simulink model "Closed_Loop_Neural_Attitude_plant_MRAC_for_roll_good"  (R2018b)
settings: Solver=VariableStepAuto  StartTime=0.0  StopTime=500  FixedStep=0.0001  RelTol=1e3  EnableMultiTasking=on
undefined symbols (not defined in the file): DiscIntNeverNeededParam
libraries: dspmtrx3 x6, neural x3, vrlib x2, sharedutil x1
CloseFcn:
  | rtwprivate ssgencode ModelCloseRequest controller
settings Model: Creator=acer  LastModifiedBy=the other guy
settings SolverCC: ZeroCrossControl=DisableAll  AutoInsertRateTranBlk=on
settings DataIOCC: LimitDataPoints=on  SaveFormat=Array  SignalLoggingSaveFormat=ModelDataLogs
settings OptimizationCC: ExpressionDepthLimit=2147483647  LifeSpan=inf
settings DebuggingCC: SaveWithParameterizedLinksMsg=none  UnderspecifiedInitializationDetection=Classic  MergeDetectMultiDrivingBlocksExec=none  SolverPrmCheckMsg=warning  FcnCallInpInsideContextMsg=warning  StateNameClashWarn=warning  SFUnexpectedBacktrackingDiag=warning  SFNoUnconditionalDefaultTransitionDiag=warning  SFExecutionAtInitializationDiag=none
settings HardwareCC: ProdBitPerPointer=32  ProdBitPerSizeT=32  ProdBitPerPtrDiffT=32  ProdLargestAtomicFloat=None  ProdIntDivRoundTo=Undefined  ProdEndianess=Unspecified  ProdWordSize=32  ProdHWDeviceType=32-bit Generic
settings ModelReferenceCC: PropagateSignalLabelsOutOfModel=off
settings SFSimCC: SimUseLocalCustomCode=off
settings RTWCC: RTWUseLocalCustomCode=off
settings CodeAppCC: StateflowObjectComments=on
settings GRTTargetCC: TargetLangStandard=C89/C90 (ANSI)  GeneratePreprocessorConditionals=Disable all  CombineOutputUpdateFcns=off  GRTInterface=on
settings ConfigComp: CovMetricSettings=dw  CovHtmlReporting=on  CovSaveCumulativeToWorkspaceVar=on  CovSaveSingleToWorkspaceVar=on  CovExternalEMLEnable=off

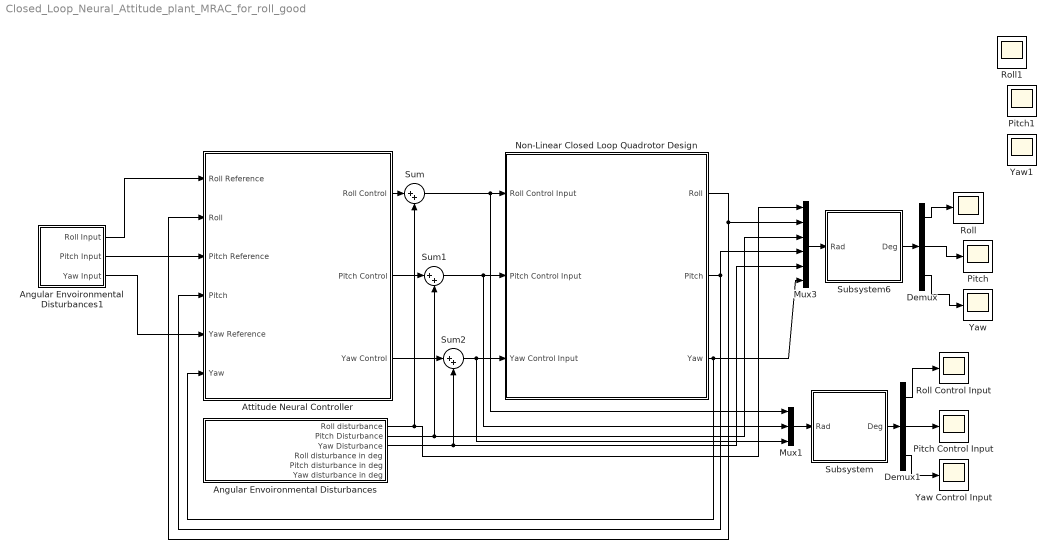
== system Closed_Loop_Neural_Attitude_plant_MRAC_for_roll_good ==
  Angular Envoironmental Disturbances : Subsystem
  Angular Envoironmental Disturbances1 : Subsystem
  Attitude Neural Controller : Subsystem
  Demux : Demux  Outputs=[2,2,2]
  Demux1 : Demux  Outputs=3
  Mux1 : Mux  Inputs=3
  Mux3 : Mux  Inputs=6
  Non-Linear Closed Loop Quadrotor Design : Subsystem
  Pitch : Scope
  Pitch Control Input : Scope
  Pitch1 : Scope
  Roll : Scope
  Roll Control Input : Scope
  Roll1 : Scope
  Subsystem : Subsystem
  Subsystem6 : Subsystem
  Sum : Sum  Inputs=|++
  Sum1 : Sum  Inputs=|++
  Sum2 : Sum  Inputs=|++
  Yaw : Scope
  Yaw Control Input : Scope
  Yaw1 : Scope
  wires:
  Non-Linear Closed Loop Quadrotor Design/1(Roll) -> Mux3/2, Attitude Neural Controller/2(Roll)
  Angular Envoironmental Disturbances1/1(Roll Input) -> Attitude Neural Controller/1(Roll Reference)
  Demux1/1 -> Roll Control Input/1
  Angular Envoironmental Disturbances1/2(Pitch Input) -> Attitude Neural Controller/3(Pitch Reference)
  Non-Linear Closed Loop Quadrotor Design/2(Pitch) -> Attitude Neural Controller/4(Pitch), Mux3/4
  Demux1/2 -> Pitch Control Input/1
  Sum1/1 -> Mux1/2, Non-Linear Closed Loop Quadrotor Design/2(Pitch Control Input)
  Sum/1 -> Mux1/1, Non-Linear Closed Loop Quadrotor Design/1(Roll Control Input)
  Sum2/1 -> Mux1/3, Non-Linear Closed Loop Quadrotor Design/3(Yaw Control Input)
  Non-Linear Closed Loop Quadrotor Design/3(Yaw) -> Attitude Neural Controller/6(Yaw), Mux3/6
  Angular Envoironmental Disturbances1/3(Yaw Input) -> Attitude Neural Controller/5(Yaw Reference)
  Demux1/3 -> Yaw Control Input/1
  Mux3/1 -> Subsystem6/1(Rad)
  Subsystem6/1(Deg) -> Demux/1
  Demux/2 -> Pitch/1
  Mux1/1 -> Subsystem/1(Rad)
  Subsystem/1(Deg) -> Demux1/1
  Attitude Neural Controller/3(Yaw Control) -> Sum2/1
  Attitude Neural Controller/2(Pitch Control) -> Sum1/1
  Attitude Neural Controller/1(Roll Control) -> Sum/1
  Demux/1 -> Roll/1
  Demux/3 -> Yaw/1
  Angular Envoironmental Disturbances/1(Roll disturbance) -> Mux3/1, Sum/2
  Angular Envoironmental Disturbances/2(Pitch Disturbance) -> Mux3/3, Sum1/2
  Angular Envoironmental Disturbances/3(Yaw Disturbance) -> Mux3/5, Sum2/2

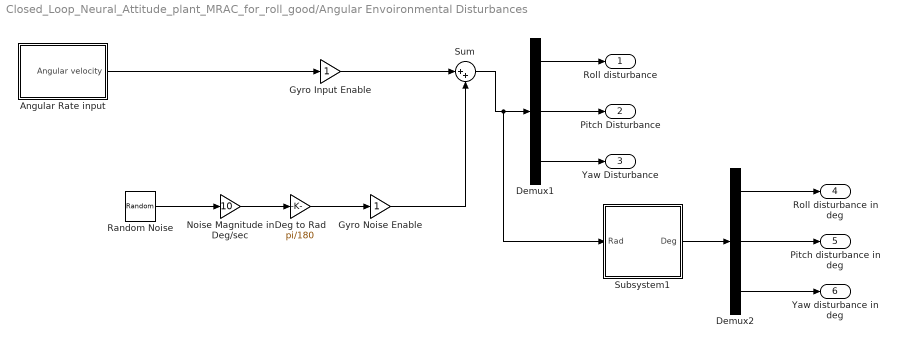
== system Closed_Loop_Neural_Attitude_plant_MRAC_for_roll_good/Angular Envoironmental Disturbances ==
  Angular Rate input : Subsystem
  Deg to Rad : Gain  Gain=pi/180
  Demux1 : Demux  Outputs=3
  Demux2 : Demux  Outputs=3
  Gyro Input Enable : Gain
  Gyro Noise Enable : Gain
  Noise Magnitude in Deg/sec : Gain  Gain=10
  Random Noise : RandomNumber  Variance=0.25  SampleTime=0
  Subsystem1 : Subsystem
  Sum : Sum  Inputs=|++
  Roll disturbance : Outport
  Pitch Disturbance : Outport  Port=2
  Yaw Disturbance : Outport  Port=3
  Roll disturbance in deg : Outport  Port=4
  Pitch disturbance in deg : Outport  Port=5
  Yaw disturbance in deg : Outport  Port=6
  wires:
  Random Noise/1 -> Noise Magnitude in Deg/sec/1
  Sum/1 -> Subsystem1/1(Rad), Demux1/1
  Gyro Noise Enable/1 -> Sum/2
  Angular Rate input/1(Angular velocity) -> Gyro Input Enable/1
  Deg to Rad/1 -> Gyro Noise Enable/1
  Noise Magnitude in Deg/sec/1 -> Deg to Rad/1
  Gyro Input Enable/1 -> Sum/1
  Demux1/1 -> Roll disturbance/1
  Demux1/2 -> Pitch Disturbance/1
  Demux1/3 -> Yaw Disturbance/1
  Subsystem1/1(Deg) -> Demux2/1
  Demux2/1 -> Roll disturbance in deg/1
  Demux2/3 -> Yaw disturbance in deg/1
  Demux2/2 -> Pitch disturbance in deg/1

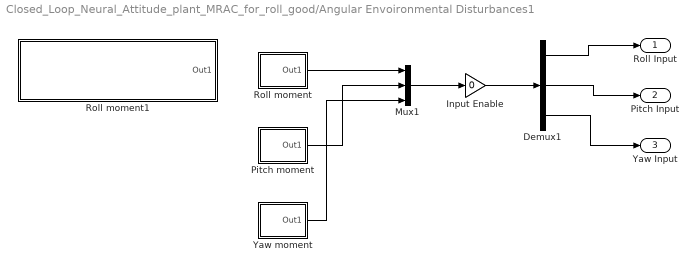
== system Closed_Loop_Neural_Attitude_plant_MRAC_for_roll_good/Angular Envoironmental Disturbances1 ==
  Demux1 : Demux  Outputs=3
  Input Enable : Gain  Gain=0
  Mux1 : Mux  Inputs=3
  Pitch moment : Subsystem  mask(timed input){t=[0 100 100 500], u=[0 0 25 25]*pi/180}
      mask prompts: t "time values:"; u "input values"
      mask Display: plot(t,u)
  Roll moment : Subsystem  mask(timed input){t=[0 200 200 500], u=[0 0 20 20]*pi/180}
      mask prompts: t "time values:"; u "input values"
      mask Display: plot(t,u)
  Roll moment1 : Subsystem  mask(timed input){t=[0 1 1 2 2 3 3 4 4 6 6 8 8 10 10 12 12 15 15 18 18 21 21 24 24 25 25 26.5 26.5 28 28 29.5 29.5 31 31 32 32 33 33 34 34 35 35 37.5, 37.5 40 40 42.5 42.5 45 45 47.5 47.5 48 48 48.5 48.5 49 49 49.5 49.5 50]*100, u=[-60 -60 60 60 60 60 -60 -60 40 40 -40 -40 -40 -40 40 40 -10 -10 10 10 10 10 -10 -10 0 0 -25 -25 25 25 25 25 -25 -25 70 70 -70 -70 -70 -70 70 70 0 0 -5 -5 5 5 5 5 -5 -5 50 50 -50 -50 -50 -50 50 50 0 0]*pi/180}
      mask prompts: t "time values:"; u "input values"
      mask Display: plot(t,u)
  Yaw moment : Subsystem  mask(timed input){t=[0 300 300 500], u=[0 0 10 10]*pi/180}
      mask prompts: t "time values:"; u "input values"
      mask Display: plot(t,u)
  Roll Input : Outport
  Pitch Input : Outport  Port=2
  Yaw Input : Outport  Port=3
  wires:
  Roll moment/1(Out1) -> Mux1/1
  Demux1/1 -> Roll Input/1
  Demux1/2 -> Pitch Input/1
  Demux1/3 -> Yaw Input/1
  Input Enable/1 -> Demux1/1
  Mux1/1 -> Input Enable/1
  Pitch moment/1(Out1) -> Mux1/2
  Yaw moment/1(Out1) -> Mux1/3

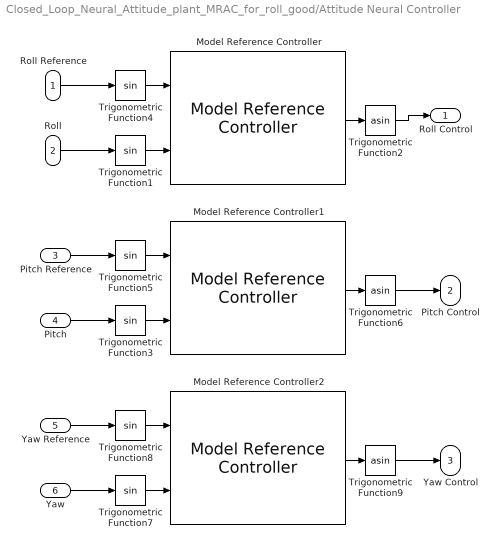
== system Closed_Loop_Neural_Attitude_plant_MRAC_for_roll_good/Attitude Neural Controller ==
  Roll Reference : Inport
  Roll : Inport  Port=2
  Pitch Reference : Inport  Port=3
  Pitch : Inport  Port=4
  Yaw Reference : Inport  Port=5
  Yaw : Inport  Port=6
  Model Reference Controller : neural/Control Systems/Model Reference Controller  Nrc=3  Nic=1  Njc=3  IW_y=[-1.0479922535678707 1.0963093533594552 0.26460365258887403;1.7732281417257523 -0.46072263125361868 0.87806211308907656;-3.1465499125506557 -0.5937319967530188 3.0204818708190166;1.0323400393569073 -0.015568814688003665 1.5371353822096789;-2.1106412934792731 0.05056036550032908 -0.14782239894507734;-1.5382119635510754 -2.1461277051649899 -0.83460054707934117;1.5622409917373894 0.78652595839841255 -0.47696768224480357;-4.9386069922881335 -0.1484318077594258 5.0391229005317655;-0.23912911789980065 0.98694261857822208 0.16515526893874477;-1.0329160606629528 -1.1960711318239752 0.90608008755680192;-0.70758561322707081 0.30837307260631891 -1.56388643801097;-0.9272694288065676 -0.91299777275763849 0.50855747578884181;-0.36702747800484953 -0.48640227843732736 0.62768503378713725;1.0337014039714969 -1.2272991141830756 0.06763723931189336;1.1463923408643808 -0.71137696889491486 -1.2171749230725455;-4.0182748202307934 -0.73468658309543133 3.0293085774035382;1.3426221912234926 1.2577183591385332 -0.090716981775017275;0.62946029749718613 -0.30092245091292902 0.016223341950540874]  IW_u=[-0.24255075731366291;0.067434596484705997;-1.0191740287778279;0.25615119174065359;-2.0112583912018533;0.22726635265696596;0.7994414553675766;-0.13599982001748542;-1.1644678637223247;0.903111284295391;1.2827580937992835;-1.3990618651287265;-1.4385363316570974;-1.7630496597549639;0.050471269965495724;0.31140070264161474;-0.24345009418100144;0.60151615384652179]  IW_r=[1.0682307206391668 1.0472325353205159 -0.2205165734628157;-1.227235953638244 -0.83152727015421402 0.91504799004562154;1.0358631742430218 -0.045817213167044693 1.7391593328913104;-1.7838274536239662 -0.05838782596051869 1.2735581550963222;1.102903994141017 0.16722990202352794 -0.77798214246003772;0.42211335887597029 0.27691864211838402 -0.44118592339890589;-0.510162099820343 0.55326224303316029 0.16224377112982155;0.92874706638522064 -0.40705446820870445 0.34285175705700727;0.5124598996000409 1.966011401792277 -1.0911026817118459;-0.70114047638361421 -0.57964817320994877 -0.19355549017515475;-0.62932233733501897 0.49900571134894584 -0.42288592192819435;0.028877083602885389 -0.30395456479522243 -1.1408313739183649;1.793567327279612 0.045223512889105914 0.5704802079274045;-0.54648636868862632 -0.74309769869801079 -0.3833340457965832;-0.44395983361533514 -1.6549080962605422 0.84302996865756374;2.5362771101602783 -0.53496813441192892 -0.54685263297492648;0.79654008306135704 -1.5868960924287974 -0.073261862756842627;0.099520489276245711 0.64658596914313327 -0.16511608967506647]  B1_c=[2.3428624787665524;-1.3936778808779784;-1.0030987335955961;-0.4509122002367793;0.051395068520306064;-1.3198924632202884;-1.2434888825122641;-1.0901675886579265;-0.72809941663907407;0.52268569615002769;-0.4469950417287647;-0.12891051881543147;-1.4934893322159866;1.2586876962327156;2.2386163377278558;-0.017545639142955476;1.4389876286566188;2.8344421537775846]  B2_c=1.2426788326263551  LW_c=[1.2470595136301488 1.1922566263341141 2.3440072598475572 -0.23302520192959994 -0.57893849507532491 0.071847335124885642 -1.5205403275306368 3.9931395156014737 -0.2292369275514731 0.51301292873069859 -0.27455950771389781 0.31671360543895116 -1.6194126272591753 -0.46530571069371418 0.55484580065879907 2.2718915739517374 -1.2298157631090092 1.337901642549306]  retraining_c=2  max_i_int=0  min_i_int=0  max_r_int=4  min_r_int=1  Ts=1  S1=5  Ni=2  Nj=2  sim_file=0  trainfun=trainlm  Use_validation=1  Use_Testing=1  Use_Inc_training=0  Use_previous_weights=1  max_i=1  min_i=-1  max_r=1  min_r=-1  sam_training=0  sam_training_c=5012  epochs=100  epochs_c=15  minp=-0.93969262078590832  maxp=0.93969262078590832  mint=-0.99823823258603839  maxt=0.93969262078590832  Normalize=0  IW=[1.1011085213037752 1.407592719906009;-0.089799928980266647 0.033955467434252179;0.19313523408982464 -0.083335702540924414;0.10317637316881607 -0.050278109734662929;0.066445533553748812 -0.2569378095580625]  LW1_2=[0.73790581738486227 0.31933069522454277;-1.1887080730231929 0.67624905941524827;0.35416604057374884 -0.34192735971607868;1.0003818253699837 -0.53447845497687374;-0.60227568611142646 -1.3054691869328516]  LW2_1=[-0.0001373472589229955 -1.4118009229408268 -1.0195237977967162 1.6886677625413407 -0.047620532601441751]  B1=[-1.5798521006707777;0.94062141810806432;0.0092618752478074249;0.39344071179103129;-2.2437335255402036]  B2=0.36905059380662364  S1c=18  Limit_output=0  min_output=0  max_output=0  Ref_file=0
      settings: SourceProductName=Deep Learning Toolbox  SourceProductBaseCode=NN
  Model Reference Controller1 : neural/Control Systems/Model Reference Controller  Nrc=3  Nic=1  Njc=3  IW_y=[-1.0479922535678707 1.0963093533594552 0.26460365258887403;1.7732281417257523 -0.46072263125361868 0.87806211308907656;-3.1465499125506557 -0.5937319967530188 3.0204818708190166;1.0323400393569073 -0.015568814688003665 1.5371353822096789;-2.1106412934792731 0.05056036550032908 -0.14782239894507734;-1.5382119635510754 -2.1461277051649899 -0.83460054707934117;1.5622409917373894 0.78652595839841255 -0.47696768224480357;-4.9386069922881335 -0.1484318077594258 5.0391229005317655;-0.23912911789980065 0.98694261857822208 0.16515526893874477;-1.0329160606629528 -1.1960711318239752 0.90608008755680192;-0.70758561322707081 0.30837307260631891 -1.56388643801097;-0.9272694288065676 -0.91299777275763849 0.50855747578884181;-0.36702747800484953 -0.48640227843732736 0.62768503378713725;1.0337014039714969 -1.2272991141830756 0.06763723931189336;1.1463923408643808 -0.71137696889491486 -1.2171749230725455;-4.0182748202307934 -0.73468658309543133 3.0293085774035382;1.3426221912234926 1.2577183591385332 -0.090716981775017275;0.62946029749718613 -0.30092245091292902 0.016223341950540874]  IW_u=[-0.24255075731366291;0.067434596484705997;-1.0191740287778279;0.25615119174065359;-2.0112583912018533;0.22726635265696596;0.7994414553675766;-0.13599982001748542;-1.1644678637223247;0.903111284295391;1.2827580937992835;-1.3990618651287265;-1.4385363316570974;-1.7630496597549639;0.050471269965495724;0.31140070264161474;-0.24345009418100144;0.60151615384652179]  IW_r=[1.0682307206391668 1.0472325353205159 -0.2205165734628157;-1.227235953638244 -0.83152727015421402 0.91504799004562154;1.0358631742430218 -0.045817213167044693 1.7391593328913104;-1.7838274536239662 -0.05838782596051869 1.2735581550963222;1.102903994141017 0.16722990202352794 -0.77798214246003772;0.42211335887597029 0.27691864211838402 -0.44118592339890589;-0.510162099820343 0.55326224303316029 0.16224377112982155;0.92874706638522064 -0.40705446820870445 0.34285175705700727;0.5124598996000409 1.966011401792277 -1.0911026817118459;-0.70114047638361421 -0.57964817320994877 -0.19355549017515475;-0.62932233733501897 0.49900571134894584 -0.42288592192819435;0.028877083602885389 -0.30395456479522243 -1.1408313739183649;1.793567327279612 0.045223512889105914 0.5704802079274045;-0.54648636868862632 -0.74309769869801079 -0.3833340457965832;-0.44395983361533514 -1.6549080962605422 0.84302996865756374;2.5362771101602783 -0.53496813441192892 -0.54685263297492648;0.79654008306135704 -1.5868960924287974 -0.073261862756842627;0.099520489276245711 0.64658596914313327 -0.16511608967506647]  B1_c=[2.3428624787665524;-1.3936778808779784;-1.0030987335955961;-0.4509122002367793;0.051395068520306064;-1.3198924632202884;-1.2434888825122641;-1.0901675886579265;-0.72809941663907407;0.52268569615002769;-0.4469950417287647;-0.12891051881543147;-1.4934893322159866;1.2586876962327156;2.2386163377278558;-0.017545639142955476;1.4389876286566188;2.8344421537775846]  B2_c=1.2426788326263551  LW_c=[1.2470595136301488 1.1922566263341141 2.3440072598475572 -0.23302520192959994 -0.57893849507532491 0.071847335124885642 -1.5205403275306368 3.9931395156014737 -0.2292369275514731 0.51301292873069859 -0.27455950771389781 0.31671360543895116 -1.6194126272591753 -0.46530571069371418 0.55484580065879907 2.2718915739517374 -1.2298157631090092 1.337901642549306]  retraining_c=2  max_i_int=0  min_i_int=0  max_r_int=4  min_r_int=1  Ts=1  S1=5  Ni=2  Nj=2  sim_file=0  trainfun=trainlm  Use_validation=1  Use_Testing=1  Use_Inc_training=0  Use_previous_weights=1  max_i=1  min_i=-1  max_r=1  min_r=-1  sam_training=0  sam_training_c=5012  epochs=100  epochs_c=15  minp=-0.93969262078590832  maxp=0.93969262078590832  mint=-0.99823823258603839  maxt=0.93969262078590832  Normalize=0  IW=[1.1011085213037752 1.407592719906009;-0.089799928980266647 0.033955467434252179;0.19313523408982464 -0.083335702540924414;0.10317637316881607 -0.050278109734662929;0.066445533553748812 -0.2569378095580625]  LW1_2=[0.73790581738486227 0.31933069522454277;-1.1887080730231929 0.67624905941524827;0.35416604057374884 -0.34192735971607868;1.0003818253699837 -0.53447845497687374;-0.60227568611142646 -1.3054691869328516]  LW2_1=[-0.0001373472589229955 -1.4118009229408268 -1.0195237977967162 1.6886677625413407 -0.047620532601441751]  B1=[-1.5798521006707777;0.94062141810806432;0.0092618752478074249;0.39344071179103129;-2.2437335255402036]  B2=0.36905059380662364  S1c=18  Limit_output=0  min_output=0  max_output=0  Ref_file=0
      settings: SourceProductName=Deep Learning Toolbox  SourceProductBaseCode=NN
  Model Reference Controller2 : neural/Control Systems/Model Reference Controller  Nrc=3  Nic=1  Njc=3  IW_y=[-1.0479922535678707 1.0963093533594552 0.26460365258887403;1.7732281417257523 -0.46072263125361868 0.87806211308907656;-3.1465499125506557 -0.5937319967530188 3.0204818708190166;1.0323400393569073 -0.015568814688003665 1.5371353822096789;-2.1106412934792731 0.05056036550032908 -0.14782239894507734;-1.5382119635510754 -2.1461277051649899 -0.83460054707934117;1.5622409917373894 0.78652595839841255 -0.47696768224480357;-4.9386069922881335 -0.1484318077594258 5.0391229005317655;-0.23912911789980065 0.98694261857822208 0.16515526893874477;-1.0329160606629528 -1.1960711318239752 0.90608008755680192;-0.70758561322707081 0.30837307260631891 -1.56388643801097;-0.9272694288065676 -0.91299777275763849 0.50855747578884181;-0.36702747800484953 -0.48640227843732736 0.62768503378713725;1.0337014039714969 -1.2272991141830756 0.06763723931189336;1.1463923408643808 -0.71137696889491486 -1.2171749230725455;-4.0182748202307934 -0.73468658309543133 3.0293085774035382;1.3426221912234926 1.2577183591385332 -0.090716981775017275;0.62946029749718613 -0.30092245091292902 0.016223341950540874]  IW_u=[-0.24255075731366291;0.067434596484705997;-1.0191740287778279;0.25615119174065359;-2.0112583912018533;0.22726635265696596;0.7994414553675766;-0.13599982001748542;-1.1644678637223247;0.903111284295391;1.2827580937992835;-1.3990618651287265;-1.4385363316570974;-1.7630496597549639;0.050471269965495724;0.31140070264161474;-0.24345009418100144;0.60151615384652179]  IW_r=[1.0682307206391668 1.0472325353205159 -0.2205165734628157;-1.227235953638244 -0.83152727015421402 0.91504799004562154;1.0358631742430218 -0.045817213167044693 1.7391593328913104;-1.7838274536239662 -0.05838782596051869 1.2735581550963222;1.102903994141017 0.16722990202352794 -0.77798214246003772;0.42211335887597029 0.27691864211838402 -0.44118592339890589;-0.510162099820343 0.55326224303316029 0.16224377112982155;0.92874706638522064 -0.40705446820870445 0.34285175705700727;0.5124598996000409 1.966011401792277 -1.0911026817118459;-0.70114047638361421 -0.57964817320994877 -0.19355549017515475;-0.62932233733501897 0.49900571134894584 -0.42288592192819435;0.028877083602885389 -0.30395456479522243 -1.1408313739183649;1.793567327279612 0.045223512889105914 0.5704802079274045;-0.54648636868862632 -0.74309769869801079 -0.3833340457965832;-0.44395983361533514 -1.6549080962605422 0.84302996865756374;2.5362771101602783 -0.53496813441192892 -0.54685263297492648;0.79654008306135704 -1.5868960924287974 -0.073261862756842627;0.099520489276245711 0.64658596914313327 -0.16511608967506647]  B1_c=[2.3428624787665524;-1.3936778808779784;-1.0030987335955961;-0.4509122002367793;0.051395068520306064;-1.3198924632202884;-1.2434888825122641;-1.0901675886579265;-0.72809941663907407;0.52268569615002769;-0.4469950417287647;-0.12891051881543147;-1.4934893322159866;1.2586876962327156;2.2386163377278558;-0.017545639142955476;1.4389876286566188;2.8344421537775846]  B2_c=1.2426788326263551  LW_c=[1.2470595136301488 1.1922566263341141 2.3440072598475572 -0.23302520192959994 -0.57893849507532491 0.071847335124885642 -1.5205403275306368 3.9931395156014737 -0.2292369275514731 0.51301292873069859 -0.27455950771389781 0.31671360543895116 -1.6194126272591753 -0.46530571069371418 0.55484580065879907 2.2718915739517374 -1.2298157631090092 1.337901642549306]  retraining_c=2  max_i_int=0  min_i_int=0  max_r_int=4  min_r_int=1  Ts=1  S1=5  Ni=2  Nj=2  sim_file=0  trainfun=trainlm  Use_validation=1  Use_Testing=1  Use_Inc_training=0  Use_previous_weights=1  max_i=1  min_i=-1  max_r=1  min_r=-1  sam_training=0  sam_training_c=5012  epochs=100  epochs_c=15  minp=-0.93969262078590832  maxp=0.93969262078590832  mint=-0.99823823258603839  maxt=0.93969262078590832  Normalize=0  IW=[1.1011085213037752 1.407592719906009;-0.089799928980266647 0.033955467434252179;0.19313523408982464 -0.083335702540924414;0.10317637316881607 -0.050278109734662929;0.066445533553748812 -0.2569378095580625]  LW1_2=[0.73790581738486227 0.31933069522454277;-1.1887080730231929 0.67624905941524827;0.35416604057374884 -0.34192735971607868;1.0003818253699837 -0.53447845497687374;-0.60227568611142646 -1.3054691869328516]  LW2_1=[-0.0001373472589229955 -1.4118009229408268 -1.0195237977967162 1.6886677625413407 -0.047620532601441751]  B1=[-1.5798521006707777;0.94062141810806432;0.0092618752478074249;0.39344071179103129;-2.2437335255402036]  B2=0.36905059380662364  S1c=18  Limit_output=0  min_output=0  max_output=0  Ref_file=0
      settings: SourceProductName=Deep Learning Toolbox  SourceProductBaseCode=NN
  Trigonometric Function{1,3..5,7..8} (6 alike) : Trigonometry
  Trigonometric Function2 : Trigonometry  Operator=asin  OutputSignalType=real
  Trigonometric Function6 : Trigonometry  Operator=asin  OutputSignalType=real
  Trigonometric Function9 : Trigonometry  Operator=asin  OutputSignalType=real
  Roll Control : Outport
  Pitch Control : Outport  Port=2
  Yaw Control : Outport  Port=3
  wires:
  Trigonometric Function5/1 -> Model Reference Controller1/1
  Model Reference Controller/1 -> Trigonometric Function2/1
  Trigonometric Function1/1 -> Model Reference Controller/2
  Trigonometric Function4/1 -> Model Reference Controller/1
  Trigonometric Function3/1 -> Model Reference Controller1/2
  Trigonometric Function6/1 -> Pitch Control/1
  Trigonometric Function2/1 -> Roll Control/1
  Model Reference Controller1/1 -> Trigonometric Function6/1
  Pitch/1 -> Trigonometric Function3/1
  Pitch Reference/1 -> Trigonometric Function5/1
  Roll Reference/1 -> Trigonometric Function4/1
  Roll/1 -> Trigonometric Function1/1
  Yaw/1 -> Trigonometric Function7/1
  Yaw Reference/1 -> Trigonometric Function8/1
  Model Reference Controller2/1 -> Trigonometric Function9/1
  Trigonometric Function7/1 -> Model Reference Controller2/2
  Trigonometric Function8/1 -> Model Reference Controller2/1
  Trigonometric Function9/1 -> Yaw Control/1

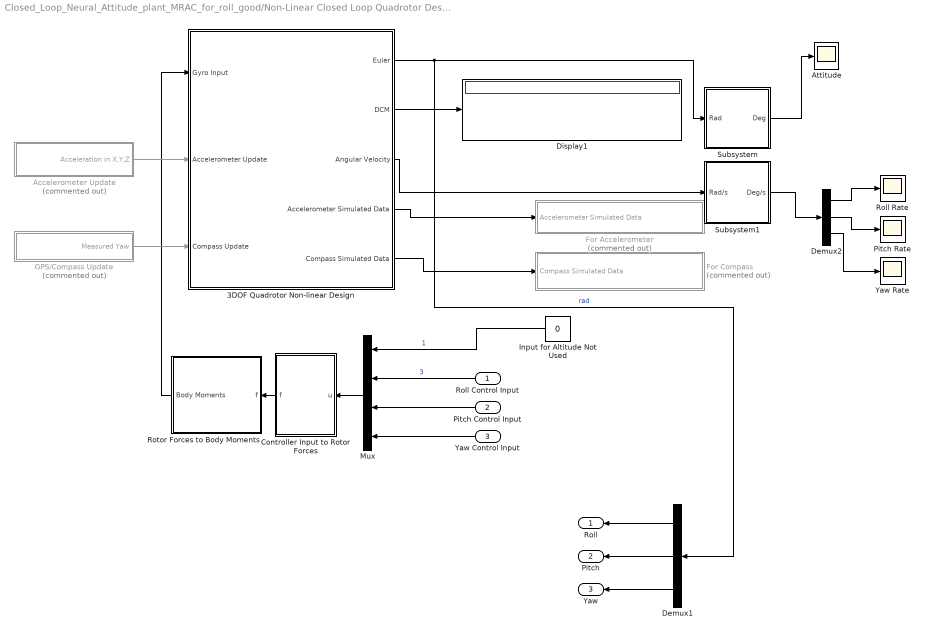
== system Closed_Loop_Neural_Attitude_plant_MRAC_for_roll_good/Non-Linear Closed Loop Quadrotor Design ==
  Roll Control Input : Inport
  Pitch Control Input : Inport  Port=2
  Yaw Control Input : Inport  Port=3
  3DOF Quadrotor Non-linear Design : Subsystem
  Accelerometer Update : Subsystem  Commented=on
  Attitude : Scope
  Controller Input to Rotor Forces : Subsystem
  Demux1 : Demux  Outputs=3
  Demux2 : Demux  Outputs=3
  Display1 : Display
  For Accelerometer : Subsystem  Commented=on
  For Compass : Subsystem  Commented=on
  GPS/Compass Update : Subsystem  Commented=on
  Input for Altitude Not Used : Constant  Value=0
  Mux : Mux
  Pitch Rate : Scope
  Roll Rate : Scope
  Rotor Forces to Body Moments : Subsystem
  Subsystem : Subsystem
  Subsystem1 : Subsystem
  Yaw Rate : Scope
  Roll : Outport
  Pitch : Outport  Port=2
  Yaw : Outport  Port=3
  wires:
  Controller Input to Rotor Forces/1(f) -> Rotor Forces to Body Moments/1(f)
  3DOF Quadrotor Non-linear Design/1(Euler) -> Demux1/1, Subsystem/1(Rad)  "rad"
  Rotor Forces to Body Moments/1(Body Moments) -> 3DOF Quadrotor Non-linear Design/1(Gyro Input)
  Accelerometer Update/1(Acceleration in X,Y,Z) -> 3DOF Quadrotor Non-linear Design/2(Accelerometer Update)
  GPS/Compass Update/1(Measured Yaw) -> 3DOF Quadrotor Non-linear Design/3(Compass Update)
  3DOF Quadrotor Non-linear Design/2(DCM) -> Display1/1
  Subsystem/1(Deg) -> Attitude/1
  Subsystem1/1(Deg/s) -> Demux2/1
  Demux2/1 -> Roll Rate/1
  Demux2/2 -> Pitch Rate/1
  Demux2/3 -> Yaw Rate/1
  3DOF Quadrotor Non-linear Design/3("Angular Velocity ") -> Subsystem1/1(Rad/s)
  3DOF Quadrotor Non-linear Design/4(Accelerometer Simulated Data) -> For Accelerometer/1(Accelerometer Simulated Data)
  3DOF Quadrotor Non-linear Design/5(Compass Simulated Data) -> For Compass/1(Compass Simulated Data)
  Input for Altitude Not Used/1 -> Mux/1  "1"
  Roll Control Input/1 -> Mux/2  "3"
  Mux/1 -> Controller Input to Rotor Forces/1(u)
  Demux1/1 -> Roll/1
  Pitch Control Input/1 -> Mux/3
  Demux1/2 -> Pitch/1
  Yaw Control Input/1 -> Mux/4
  Demux1/3 -> Yaw/1

== system Closed_Loop_Neural_Attitude_plant_MRAC_for_roll_good/Subsystem ==
  Rad : Inport
  Constant : Constant  Value=180/pi
  Product1 : Product  RndMeth=Zero
  Deg : Outport
  wires:
  Constant/1 -> Product1/2
  Rad/1 -> Product1/1
  Product1/1 -> Deg/1

== system Closed_Loop_Neural_Attitude_plant_MRAC_for_roll_good/Subsystem6 ==
  Rad : Inport
  Constant : Constant  Value=180/pi
  Product1 : Product  RndMeth=Zero
  Deg : Outport
  wires:
  Constant/1 -> Product1/2
  Rad/1 -> Product1/1
  Product1/1 -> Deg/1

== system Closed_Loop_Neural_Attitude_plant_MRAC_for_roll_good/Angular Envoironmental Disturbances/Angular Rate input ==
  Mux : Mux  Inputs=3
  Pitch moment : Subsystem  mask(timed input){t=[0 100 100 200 200 300 300 400 400 500]-50, u=[0 0 40 40 0 0 -40 -40 0 0]*pi/180}
      mask prompts: t "time values:"; u "input values"
      mask Display: plot(t,u)
  Roll moment : Subsystem  mask(timed input){t=[0 150 150 250 250 350 350 450 450 500]-50, u=[0 0 30 30 0 0 -30 -30 0 0]*pi/180}
      mask prompts: t "time values:"; u "input values"
      mask Display: plot(t,u)
  Yaw moment : Subsystem  mask(timed input){t=[0 225 225 325 325 425 425 525 525 550]-50, u=[0 0 45 45 0 0 -45 -45 0 0]*pi/180}
      mask prompts: t "time values:"; u "input values"
      mask Display: plot(t,u)
  Angular velocity : Outport
  wires:
  Roll moment/1(Out1) -> Mux/1
  Pitch moment/1(Out1) -> Mux/2
  Yaw moment/1(Out1) -> Mux/3
  Mux/1 -> Angular velocity/1

== system Closed_Loop_Neural_Attitude_plant_MRAC_for_roll_good/Angular Envoironmental Disturbances/Subsystem1 ==
  Rad : Inport
  Constant : Constant  Value=180/pi
  Product1 : Product  RndMeth=Zero
  Deg : Outport
  wires:
  Constant/1 -> Product1/2
  Rad/1 -> Product1/1
  Product1/1 -> Deg/1

== system Closed_Loop_Neural_Attitude_plant_MRAC_for_roll_good/Angular Envoironmental Disturbances1/Pitch moment ==
  From Workspace : FromWorkspace  VariableName=[t',u']  SampleTime=0
  Out1 : Outport
  wires:
  From Workspace/1 -> Out1/1

== system Closed_Loop_Neural_Attitude_plant_MRAC_for_roll_good/Angular Envoironmental Disturbances1/Roll moment ==
  From Workspace : FromWorkspace  VariableName=[t',u']  SampleTime=0
  Out1 : Outport
  wires:
  From Workspace/1 -> Out1/1

== system Closed_Loop_Neural_Attitude_plant_MRAC_for_roll_good/Angular Envoironmental Disturbances1/Roll moment1 ==
  From Workspace : FromWorkspace  VariableName=[t',u']  SampleTime=0
  Out1 : Outport
  wires:
  From Workspace/1 -> Out1/1

== system Closed_Loop_Neural_Attitude_plant_MRAC_for_roll_good/Angular Envoironmental Disturbances1/Yaw moment ==
  From Workspace : FromWorkspace  VariableName=[t',u']  SampleTime=0
  Out1 : Outport
  wires:
  From Workspace/1 -> Out1/1

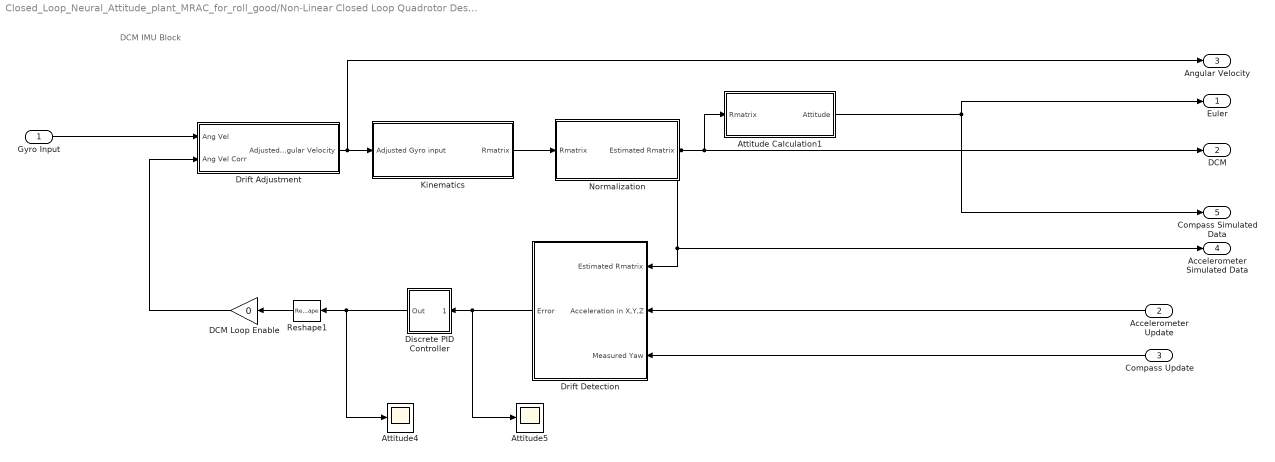
== system Closed_Loop_Neural_Attitude_plant_MRAC_for_roll_good/Non-Linear Closed Loop Quadrotor Design/3DOF Quadrotor Non-linear Design ==
  note: DCM IMU Block
  Gyro Input : Inport
  Accelerometer Update : Inport  Port=2
  Compass Update : Inport  Port=3
  Attitude Calculation1 : Subsystem
  Attitude4 : Scope
  Attitude5 : Scope
  DCM Loop Enable : Gain  Gain=0
  Discrete PID Controller : Subsystem  AncestorBlock=|  DialogController=POWERSYS.PowerSysDialog  mask(Discrete PID Controller){Kp=5, Ki=2, Kd=0, TcD=0, Par_Limits=[1e6 -1e6], Init=0, Ts=1}
      | powerlib_extras/Discrete 
      | Control Blocks/Discrete
      | PID Controller
      mask prompts: Kp "Proportional gain (Kp):"; Ki "Integral gain (Ki):"; Kd "Derivative gain (Kd):"; TcD "Time constant for derivative (s):"; Par_Limits "Output limits: [ Upper   Lower ]"; Init "Output initial value:"; Ts "Sample time:"
      mask help: This block implements a discrete PID controller.
      mask init:
      | UpperLimit=Par_Limits(1);
      | LowerLimit=Par_Limits(2);
      | power_initmask();
      mask Help: This block is part of a subset of blocks in the Extras library that does not have documentation associated with it, other than the block mask description.
      mask Display: disp('PID');
  Drift Adjustment : Subsystem
  Drift Detection : Subsystem
  Kinematics : Subsystem
  Normalization : Subsystem
  Reshape1 : Reshape  OutputDimensionality=Column vector (2-D)
  Euler : Outport
  DCM : Outport  Port=2
  "Angular Velocity " : Outport  Port=3
  Accelerometer Simulated Data : Outport  Port=4
  Compass Simulated Data : Outport  Port=5
  wires:
  Attitude Calculation1/1(Attitude) -> Euler/1, Compass Simulated Data/1
  Drift Adjustment/1(Adjusted Angular Velocity) -> "Angular Velocity "/1, Kinematics/1(Adjusted Gyro input)
  Gyro Input/1 -> Drift Adjustment/1(Ang Vel)
  Compass Update/1 -> Drift Detection/3(Measured Yaw)
  Drift Detection/1(Error) -> Attitude5/1, Discrete PID Controller/1(Error)
  Discrete PID Controller/1(Out) -> Attitude4/1, Reshape1/1
  Accelerometer Update/1 -> Drift Detection/2(Acceleration in X,Y,Z)
  Reshape1/1 -> DCM Loop Enable/1
  DCM Loop Enable/1 -> Drift Adjustment/2(Ang Vel Corr)
  Normalization/1(Estimated Rmatrix) -> Accelerometer Simulated Data/1, Drift Detection/1(Estimated Rmatrix), Attitude Calculation1/1(Rmatrix), DCM/1
  Kinematics/1(Rmatrix) -> Normalization/1(Rmatrix)

== system Closed_Loop_Neural_Attitude_plant_MRAC_for_roll_good/Non-Linear Closed Loop Quadrotor Design/Accelerometer Update ==
  Attitude2 : Scope
  From File : FromFile  FileName=acceleration_from_simulink  SampleTime=0
  Acceleration in X,Y,Z : Outport
  wires:
  From File/1 -> Attitude2/1, Acceleration in X,Y,Z/1

== system Closed_Loop_Neural_Attitude_plant_MRAC_for_roll_good/Non-Linear Closed Loop Quadrotor Design/Controller Input to Rotor Forces ==
  u : Inport
  Matrix Multiply : Product  Multiplication=Matrix(*)
  inv(plant_model) : Constant  Value=|  VectorParams1D=off
      | [  -0.2500         0   -0.5000   -0.2500
      |  ;  -0.2500   -0.5000         0    0.2500
      |   ; -0.2500         0    0.5000   -0.2500
      |   ; -0.2500    0.5000         0    0.2500
      | ]
  f : Outport
  wires:
  inv(plant_model)/1 -> Matrix Multiply/1
  Matrix Multiply/1 -> f/1
  u/1 -> Matrix Multiply/2

== system Closed_Loop_Neural_Attitude_plant_MRAC_for_roll_good/Non-Linear Closed Loop Quadrotor Design/For Accelerometer ==
  Accelerometer Simulated Data : Inport
  Embedded MATLAB Function1 : MATLAB Function  TreatAsAtomicUnit=on
  For acceleration : ToFile  Filename=acceleration_from_simulink.mat
  Mux : Mux  Inputs=3
  wires:
  Embedded MATLAB Function1/1(accel_x) -> Mux/1
  Embedded MATLAB Function1/3(accel_z) -> Mux/3
  Mux/1 -> For acceleration/1
  Embedded MATLAB Function1/2(accel_y) -> Mux/2
  Accelerometer Simulated Data/1 -> Embedded MATLAB Function1/1(R_t_n)

== system Closed_Loop_Neural_Attitude_plant_MRAC_for_roll_good/Non-Linear Closed Loop Quadrotor Design/For Compass ==
  Compass Simulated Data : Inport
  Demux1 : Demux  Outputs=3
  For Compass : ToFile  Filename=yaw_from_simulink
  Terminator1 : Terminator
  Terminator2 : Terminator
  wires:
  Compass Simulated Data/1 -> Demux1/1
  Demux1/2 -> Terminator2/1
  Demux1/1 -> Terminator1/1
  Demux1/3 -> For Compass/1

== system Closed_Loop_Neural_Attitude_plant_MRAC_for_roll_good/Non-Linear Closed Loop Quadrotor Design/GPS//Compass Update ==
  Attitude3 : Scope
  GPS/Compass Update : FromFile  FileName=yaw_from_simulink  SampleTime=0
  Subsystem2 : Subsystem
  Measured Yaw : Outport
  wires:
  GPS/Compass Update/1 -> Subsystem2/1(Rad), Measured Yaw/1
  Subsystem2/1(Deg) -> Attitude3/1

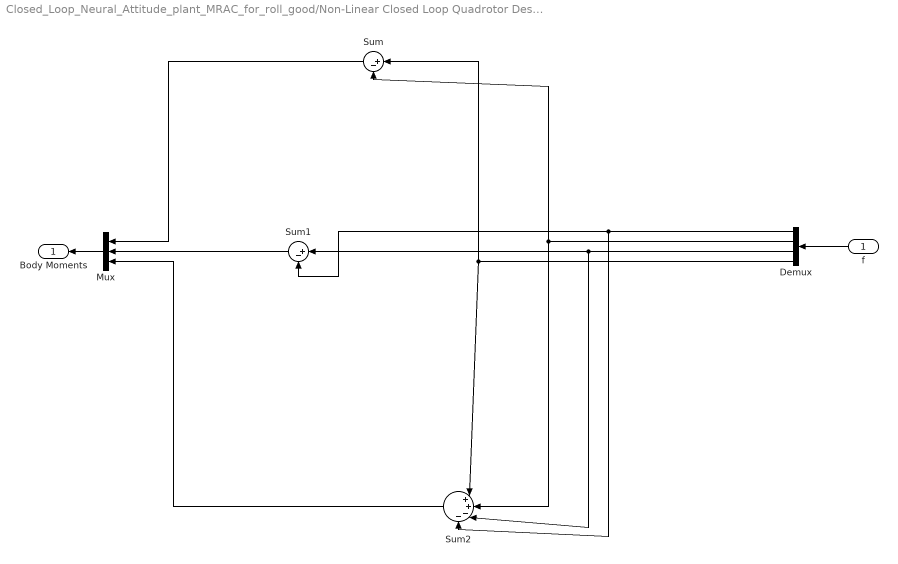
== system Closed_Loop_Neural_Attitude_plant_MRAC_for_roll_good/Non-Linear Closed Loop Quadrotor Design/Rotor Forces to Body Moments ==
  f : Inport
  Demux : Demux
  Mux : Mux  Inputs=3
  Sum : Sum  Inputs=|+-
  Sum1 : Sum  Inputs=|+-
  Sum2 : Sum  Inputs=|++--
  Body Moments : Outport
  wires:
  Sum/1 -> Mux/1
  Sum1/1 -> Mux/2
  Sum2/1 -> Mux/3
  f/1 -> Demux/1
  Mux/1 -> Body Moments/1
  Demux/1 -> Sum1/2, Sum2/4
  Demux/2 -> Sum2/2, Sum/2
  Demux/3 -> Sum1/1, Sum2/3
  Demux/4 -> Sum2/1, Sum/1

== system Closed_Loop_Neural_Attitude_plant_MRAC_for_roll_good/Non-Linear Closed Loop Quadrotor Design/Subsystem ==
  Rad : Inport
  Constant : Constant  Value=180/pi
  Product1 : Product  RndMeth=Zero
  Deg : Outport
  wires:
  Constant/1 -> Product1/2
  Rad/1 -> Product1/1
  Product1/1 -> Deg/1

== system Closed_Loop_Neural_Attitude_plant_MRAC_for_roll_good/Non-Linear Closed Loop Quadrotor Design/Subsystem1 ==
  Rad/s : Inport
  Constant : Constant  Value=180/pi
  Product1 : Product  RndMeth=Zero
  Deg/s : Outport
  wires:
  Constant/1 -> Product1/2
  Rad/s/1 -> Product1/1
  Product1/1 -> Deg/s/1

== system Closed_Loop_Neural_Attitude_plant_MRAC_for_roll_good/Angular Envoironmental Disturbances/Angular Rate input/Pitch moment ==
  From Workspace : FromWorkspace  VariableName=[t',u']  SampleTime=0
  Out1 : Outport
  wires:
  From Workspace/1 -> Out1/1

== system Closed_Loop_Neural_Attitude_plant_MRAC_for_roll_good/Angular Envoironmental Disturbances/Angular Rate input/Roll moment ==
  From Workspace : FromWorkspace  VariableName=[t',u']  SampleTime=0
  Out1 : Outport
  wires:
  From Workspace/1 -> Out1/1

== system Closed_Loop_Neural_Attitude_plant_MRAC_for_roll_good/Angular Envoironmental Disturbances/Angular Rate input/Yaw moment ==
  From Workspace : FromWorkspace  VariableName=[t',u']  SampleTime=0
  Out1 : Outport
  wires:
  From Workspace/1 -> Out1/1

== system Closed_Loop_Neural_Attitude_plant_MRAC_for_roll_good/Non-Linear Closed Loop Quadrotor Design/3DOF Quadrotor Non-linear Design/Attitude Calculation1 ==
  Rmatrix : Inport
  Embedded MATLAB Function1 : MATLAB Function  TreatAsAtomicUnit=on
  Mux : Mux  Inputs=3
  Attitude : Outport
  wires:
  Embedded MATLAB Function1/1(Roll) -> Mux/1
  Mux/1 -> Attitude/1
  Rmatrix/1 -> Embedded MATLAB Function1/1(R_mat)
  Embedded MATLAB Function1/2(Pitch) -> Mux/2
  Embedded MATLAB Function1/3(Yaw) -> Mux/3

== system Closed_Loop_Neural_Attitude_plant_MRAC_for_roll_good/Non-Linear Closed Loop Quadrotor Design/3DOF Quadrotor Non-linear Design/Discrete PID Controller ==
  note: Pierre Giroux, Gilbert Sybille
      | Power System Simulation Laboratory
      | IREQ, Hydro-Quebc
  note: Discrete PID Controller
  Error : Inport
  Discrete-Time Integrator : DiscreteIntegrator  InitialCondition=Init  SampleTime=Ts  LimitOutput=on  UpperSaturationLimit=UpperLimit  LowerSaturationLimit=LowerLimit  ICPrevOutput=DiscIntNeverNeededParam  ICPrevScaledInput=DiscIntNeverNeededParam
  Kp4 : Gain  Gain=Kp  SaturateOnIntegerOverflow=on  OutDataTypeStr=Inherit: Same as input  ParamDataTypeStr=Inherit: Same as input
  Kp5 : Gain  Gain=Ki  SaturateOnIntegerOverflow=on  OutDataTypeStr=Inherit: Same as input  ParamDataTypeStr=Inherit: Same as input
  Saturation2 : Saturate  UpperLimit=UpperLimit  LowerLimit=LowerLimit
  Sum6 : Sum  SaturateOnIntegerOverflow=on  InputSameDT=on  OutDataTypeStr=Inherit: Same as first input
  Out : Outport  InitialOutput=0
  wires:
  Error/1 -> Kp4/1, Kp5/1
  Sum6/1 -> Saturation2/1
  Kp5/1 -> Discrete-Time Integrator/1
  Kp4/1 -> Sum6/1
  Discrete-Time Integrator/1 -> Sum6/2
  Saturation2/1 -> Out/1

== system Closed_Loop_Neural_Attitude_plant_MRAC_for_roll_good/Non-Linear Closed Loop Quadrotor Design/3DOF Quadrotor Non-linear Design/Drift Adjustment ==
  Ang Vel : Inport
  Ang Vel Corr : Inport  Port=2
  Sum : Sum  Inputs=|+-
  Adjusted Angular Velocity : Outport
  wires:
  Ang Vel/1 -> Sum/1
  Sum/1 -> Adjusted Angular Velocity/1
  Ang Vel Corr/1 -> Sum/2

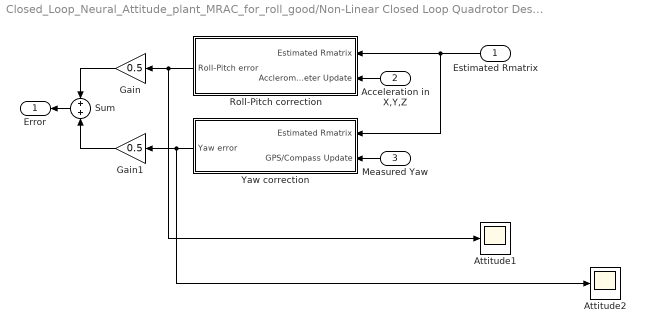
== system Closed_Loop_Neural_Attitude_plant_MRAC_for_roll_good/Non-Linear Closed Loop Quadrotor Design/3DOF Quadrotor Non-linear Design/Drift Detection ==
  Estimated Rmatrix : Inport
  Acceleration in X,Y,Z : Inport  Port=2
  Measured Yaw : Inport  Port=3
  Attitude1 : Scope
  Attitude2 : Scope
  Gain : Gain  Gain=0.5
  Gain1 : Gain  Gain=0.5
  Roll-Pitch correction : Subsystem
  Sum : Sum
  Yaw correction : Subsystem
  Error : Outport
  wires:
  Roll-Pitch correction/1(Roll-Pitch error) -> Attitude1/1, Gain/1
  Yaw correction/1(Yaw error) -> Attitude2/1, Gain1/1
  Estimated Rmatrix/1 -> Roll-Pitch correction/1(Estimated Rmatrix), Yaw correction/1(Estimated Rmatrix)
  Acceleration in X,Y,Z/1 -> Roll-Pitch correction/2(Acclerometer Update)
  Measured Yaw/1 -> Yaw correction/2(GPS/Compass Update)
  Sum/1 -> Error/1
  Gain/1 -> Sum/1
  Gain1/1 -> Sum/2

== system Closed_Loop_Neural_Attitude_plant_MRAC_for_roll_good/Non-Linear Closed Loop Quadrotor Design/3DOF Quadrotor Non-linear Design/Kinematics ==
  Adjusted Gyro input : Inport
  Demux : Demux  Outputs=3
  Embedded MATLAB Function : MATLAB Function  TreatAsAtomicUnit=on
  Memory : Memory
  Rmatrix : Outport
  wires:
  Demux/1 -> Embedded MATLAB Function/1(R_rate)
  Demux/2 -> Embedded MATLAB Function/2(P_rate)
  Demux/3 -> Embedded MATLAB Function/3(Y_rate)
  Embedded MATLAB Function/1(R_t) -> Memory/1, Rmatrix/1
  Memory/1 -> Embedded MATLAB Function/4(R_t_i)
  Adjusted Gyro input/1 -> Demux/1

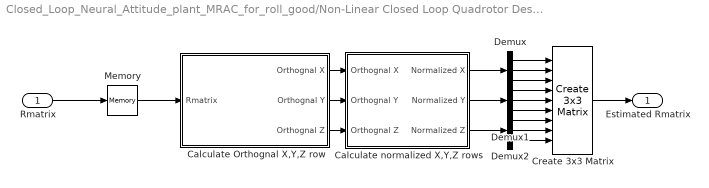
== system Closed_Loop_Neural_Attitude_plant_MRAC_for_roll_good/Non-Linear Closed Loop Quadrotor Design/3DOF Quadrotor Non-linear Design/Normalization ==
  Rmatrix : Inport
  Calculate Orthognal X,Y,Z row : Subsystem
  Calculate normalized X,Y,Z rows : Subsystem
  Create 3x3 Matrix : sharedutil/Create 3x3 Matrix  aMode=aMode
  Demux : Demux  Outputs=3
  Demux1 : Demux  Outputs=3
  Demux2 : Demux  Outputs=3
  Memory : Memory
  Estimated Rmatrix : Outport
  wires:
  Calculate normalized X,Y,Z rows/1(Normalized X) -> Demux/1
  Calculate normalized X,Y,Z rows/2(Normalized Y) -> Demux1/1
  Calculate normalized X,Y,Z rows/3(Normalized Z) -> Demux2/1
  Demux/1 -> Create 3x3 Matrix/1
  Demux/2 -> Create 3x3 Matrix/2
  Demux/3 -> Create 3x3 Matrix/3
  Demux1/1 -> Create 3x3 Matrix/4
  Demux1/2 -> Create 3x3 Matrix/5
  Demux1/3 -> Create 3x3 Matrix/6
  Demux2/1 -> Create 3x3 Matrix/7
  Demux2/2 -> Create 3x3 Matrix/8
  Demux2/3 -> Create 3x3 Matrix/9
  Calculate Orthognal X,Y,Z row/1(Orthognal X) -> Calculate normalized X,Y,Z rows/1(Orthognal X)
  Calculate Orthognal X,Y,Z row/2(Orthognal Y) -> Calculate normalized X,Y,Z rows/2(Orthognal Y)
  Calculate Orthognal X,Y,Z row/3(Orthognal Z) -> Calculate normalized X,Y,Z rows/3(Orthognal Z)
  Rmatrix/1 -> Memory/1
  Create 3x3 Matrix/1 -> Estimated Rmatrix/1
  Memory/1 -> Calculate Orthognal X,Y,Z row/1(Rmatrix)

== system Closed_Loop_Neural_Attitude_plant_MRAC_for_roll_good/Non-Linear Closed Loop Quadrotor Design/GPS//Compass Update/Subsystem2 ==
  Rad : Inport
  Constant : Constant  Value=180/pi
  Product1 : Product  RndMeth=Zero
  Deg : Outport
  wires:
  Constant/1 -> Product1/2
  Rad/1 -> Product1/1
  Product1/1 -> Deg/1

== system Closed_Loop_Neural_Attitude_plant_MRAC_for_roll_good/Non-Linear Closed Loop Quadrotor Design/3DOF Quadrotor Non-linear Design/Drift Detection/Roll-Pitch correction ==
  Estimated Rmatrix : Inport
  Acclerometer Update : Inport  Port=2
  Cross Product : vrlib/Utilities/Cross Product
      settings: SourceProductBaseCode=VR
  Row 3 selection : dspmtrx3/Submatrix  RowSpan=One row  RowStartMode=Last  RowStartIndex=1  RowEndMode=Last  RowEndIndex=1  ColSpan=All columns  ColStartMode=Last  ColStartIndex=1  ColEndMode=Last  ColEndIndex=1
  Roll-Pitch error : Outport
  wires:
  Estimated Rmatrix/1 -> Row 3 selection/1
  Cross Product/1 -> Roll-Pitch error/1
  Acclerometer Update/1 -> Cross Product/2
  Row 3 selection/1 -> Cross Product/1

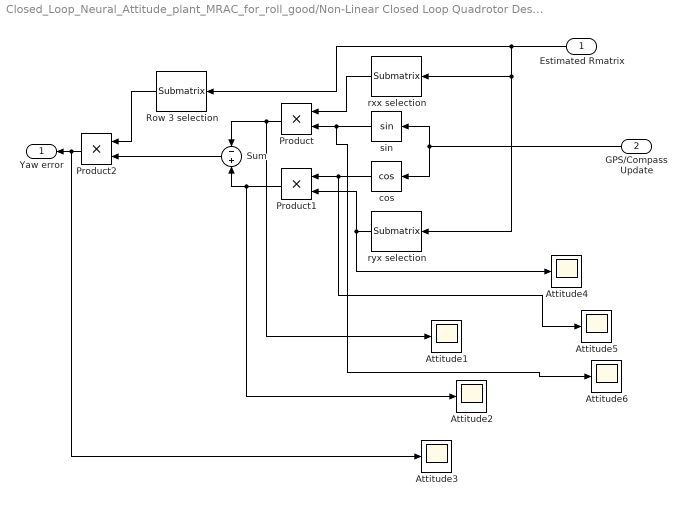
== system Closed_Loop_Neural_Attitude_plant_MRAC_for_roll_good/Non-Linear Closed Loop Quadrotor Design/3DOF Quadrotor Non-linear Design/Drift Detection/Yaw correction ==
  Estimated Rmatrix : Inport
  GPS/Compass Update : Inport  Port=2
  Attitude{1..6} (6 alike) : Scope
  Product : Product  RndMeth=Zero
  Product1 : Product  RndMeth=Zero
  Product2 : Product  RndMeth=Zero
  Row 3 selection : dspmtrx3/Submatrix  RowSpan=One row  RowStartMode=Last  RowStartIndex=1  RowEndMode=Last  RowEndIndex=1  ColSpan=All columns  ColStartMode=First  ColStartIndex=1  ColEndMode=Last  ColEndIndex=1
  Sum : Sum  Inputs=-+
  cos : Trigonometry  Operator=cos
  rxx selection : dspmtrx3/Submatrix  RowSpan=One row  RowStartMode=First  RowStartIndex=1  RowEndMode=Last  RowEndIndex=1  ColSpan=One column  ColStartMode=First  ColStartIndex=1  ColEndMode=Last  ColEndIndex=1
  ryx selection : dspmtrx3/Submatrix  RowSpan=One row  RowStartMode=Middle  RowStartIndex=1  RowEndMode=Last  RowEndIndex=1  ColSpan=One column  ColStartMode=First  ColStartIndex=1  ColEndMode=Last  ColEndIndex=1
  sin : Trigonometry
  Yaw error : Outport
  wires:
  rxx selection/1 -> Product/1
  sin/1 -> Attitude6/1, Product/2
  ryx selection/1 -> Product1/2, Attitude4/1
  cos/1 -> Attitude5/1, Product1/1
  Product/1 -> Attitude1/1, Sum/1
  Product1/1 -> Attitude2/1, Sum/2
  Row 3 selection/1 -> Product2/1
  Sum/1 -> Product2/2
  Estimated Rmatrix/1 -> Row 3 selection/1, ryx selection/1, rxx selection/1
  GPS/Compass Update/1 -> cos/1, sin/1
  Product2/1 -> Attitude3/1, Yaw error/1

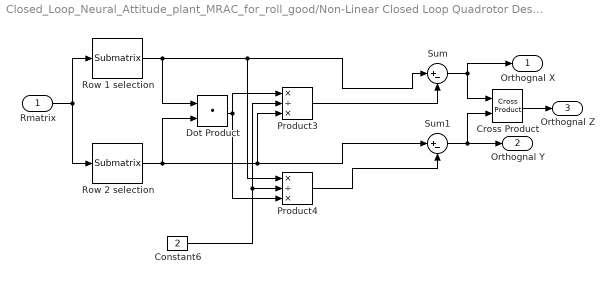
== system Closed_Loop_Neural_Attitude_plant_MRAC_for_roll_good/Non-Linear Closed Loop Quadrotor Design/3DOF Quadrotor Non-linear Design/Normalization/Calculate Orthognal X,Y,Z row ==
  Rmatrix : Inport
  Constant6 : Constant  Value=2
  Cross Product : vrlib/Utilities/Cross Product
      settings: SourceProductBaseCode=VR
  Dot Product : DotProduct  InputSameDT=on  OutDataTypeStr=Inherit: Inherit via internal rule
  Product3 : Product  Inputs=*/*  RndMeth=Zero
  Product4 : Product  Inputs=*/*  RndMeth=Zero
  Row 1 selection : dspmtrx3/Submatrix  RowSpan=One row  RowStartMode=First  RowStartIndex=1  RowEndMode=Last  RowEndIndex=1  ColSpan=All columns  ColStartMode=First  ColStartIndex=1  ColEndMode=Last  ColEndIndex=1
  Row 2 selection : dspmtrx3/Submatrix  RowSpan=One row  RowStartMode=Middle  RowStartIndex=1  RowEndMode=Last  RowEndIndex=1  ColSpan=All columns  ColStartMode=First  ColStartIndex=1  ColEndMode=Last  ColEndIndex=1
  Sum : Sum  Inputs=|+-
  Sum1 : Sum  Inputs=|+-
  Orthognal X : Outport
  Orthognal Y : Outport  Port=2
  Orthognal Z : Outport  Port=3
  wires:
  Sum/1 -> Cross Product/1, Orthognal X/1
  Sum1/1 -> Cross Product/2, Orthognal Y/1
  Row 1 selection/1 -> Product4/1, Sum/1, Dot Product/1
  Row 2 selection/1 -> Product3/3, Sum1/1, Dot Product/2
  Constant6/1 -> Product3/2, Product4/2
  Product3/1 -> Sum/2
  Product4/1 -> Sum1/2
  Cross Product/1 -> Orthognal Z/1
  Rmatrix/1 -> Row 1 selection/1, Row 2 selection/1
  Dot Product/1 -> Product4/3, Product3/1

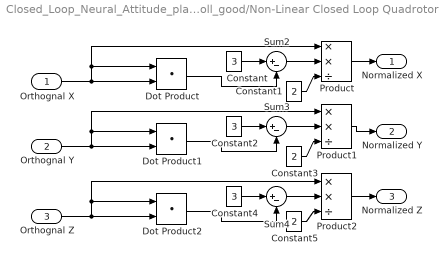
== system Closed_Loop_Neural_Attitude_plant_MRAC_for_roll_good/Non-Linear Closed Loop Quadrotor Design/3DOF Quadrotor Non-linear Design/Normalization/Calculate normalized X,Y,Z rows ==
  Orthognal X : Inport
  Orthognal Y : Inport  Port=2
  Orthognal Z : Inport  Port=3
  Constant : Constant  Value=3
  Constant1 : Constant  Value=2
  Constant2 : Constant  Value=3
  Constant3 : Constant  Value=2
  Constant4 : Constant  Value=3
  Constant5 : Constant  Value=2
  Dot Product : DotProduct  InputSameDT=on  OutDataTypeStr=Inherit: Inherit via internal rule
  Dot Product1 : DotProduct  InputSameDT=on  OutDataTypeStr=Inherit: Inherit via internal rule
  Dot Product2 : DotProduct  InputSameDT=on  OutDataTypeStr=Inherit: Inherit via internal rule
  Product : Product  Inputs=**/  RndMeth=Zero
  Product1 : Product  Inputs=**/  RndMeth=Zero
  Product2 : Product  Inputs=**/  RndMeth=Zero
  Sum2 : Sum  Inputs=|+-
  Sum3 : Sum  Inputs=|+-
  Sum4 : Sum  Inputs=|+-
  Normalized X : Outport
  Normalized Y : Outport  Port=2
  Normalized Z : Outport  Port=3
  wires:
  Constant/1 -> Sum2/1
  Sum2/1 -> Product/2
  Constant1/1 -> Product/3
  Constant2/1 -> Sum3/1
  Sum3/1 -> Product1/2
  Constant3/1 -> Product1/3
  Constant4/1 -> Sum4/1
  Sum4/1 -> Product2/2
  Constant5/1 -> Product2/3
  Product/1 -> Normalized X/1
  Product1/1 -> Normalized Y/1
  Product2/1 -> Normalized Z/1
  Orthognal X/1 -> Dot Product/2, Dot Product/1, Product/1
  Dot Product/1 -> Sum2/2
  Orthognal Y/1 -> Dot Product1/2, Dot Product1/1, Product1/1
  Dot Product1/1 -> Sum3/2
  Orthognal Z/1 -> Dot Product2/2, Dot Product2/1, Product2/1
  Dot Product2/1 -> Sum4/2

== matlab function Closed_Loop_Neural_Attitude_plant_MRAC_for_roll_good/Non-Linear Closed Loop Quadrotor Design/3DOF Quadrotor Non-linear Design/Kinematics/Embedded MATLAB Function ==
  data: R_rate input; R_t output; P_rate input; Y_rate input; R_t_i input
function R_t= fcn(R_rate,P_rate,Y_rate,R_t_i)
%--------------------Calculate Change in Rmatrix-------------------
dt=0.01;
a11=1;
a22=1;
a33=1;
a12=-Y_rate*dt;
a13=P_rate*dt;
a21=Y_rate*dt;
a23=-R_rate*dt;
a31=-P_rate*dt;
a32=R_rate*dt;
R_dt=[a11 a12 a13;a21 a22 a23;a31 a32 a33];
%--------------------Update Rmatrix-------------------------------
if (det(R_t_i)==0)
    R_t=[1 0 0;0 1 0;0 0 1];
else R_t=R_t_i;
end

R_t=R_t*R_dt;
% R_t=R_dt*R_t;

== matlab function Closed_Loop_Neural_Attitude_plant_MRAC_for_roll_good/Non-Linear Closed Loop Quadrotor Design/For Accelerometer/Embedded MATLAB Function1 ==
  data: R_t_n input; accel_x output; accel_y output; accel_z output
function [accel_x,accel_y,accel_z] = fcn(R_t_n)
Roll = atan2(R_t_n(3,2),R_t_n(3,3));
acc_x=(9.8160*R_t_n(3,1));     %at the moment we are calculating
acc_y=(9.8160*sin(Roll));     %gravity vector in X,Y,Z directions
acc_z=sqrt(9.8160^2-(acc_y)^2-(acc_x)^2);
accel_x=acc_x/sqrt(acc_x^2+acc_y^2+acc_z^2);
accel_y=acc_y/sqrt(acc_x^2+acc_y^2+acc_z^2);
accel_z=acc_z/sqrt(acc_x^2+acc_y^2+acc_z^2);

== matlab function Closed_Loop_Neural_Attitude_plant_MRAC_for_roll_good/Non-Linear Closed Loop Quadrotor Design/3DOF Quadrotor Non-linear Design/Attitude Calculation1/Embedded MATLAB Function1 ==
  data: R_mat input; Roll output; Pitch output; Yaw output
function [Roll, Pitch, Yaw] = asin(R_mat)
% Roll = atan2(u(2,3),u(3,3));
% Pitch=-asin(u(1,3));
% Yaw=atan2(u(1,2),u(1,1));
Roll = atan2(R_mat(3,2),R_mat(3,3));
Pitch=-asin(R_mat(3,1));
Yaw=atan2(R_mat(2,1),R_mat(1,1));
